simulink model "Hunt_crossley"  (Simulink 10.1)
settings: Solver=ode3  StartTime=0.0  StopTime=25  FixedStep=0.001  RelTol=1e-3  EnableMultiTasking=on
undefined symbols (not defined in the file): sigbuilder_block
libraries: simulink x3
settings Model: Creator=x  LastModifiedBy=pedram
settings DataIOCC: LimitDataPoints=on
settings OptimizationCC: ExpressionDepthLimit=2147483647
settings DebuggingCC: SolverPrmCheckMsg=warning  StateNameClashWarn=warning
settings GRTTargetCC: CombineOutputUpdateFcns=on  GRTInterface=off

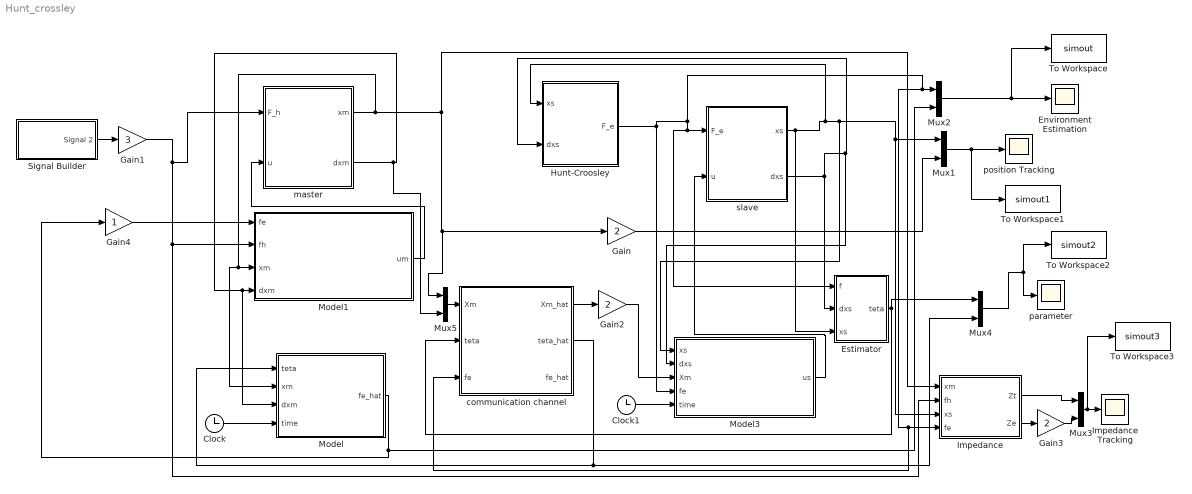
== system Hunt_crossley ==
  Clock : Clock
  Clock1 : Clock
  Environment Estimation : Scope
  Estimator : Subsystem
  Gain : Gain  Gain=2
  Gain1 : Gain  Gain=3
  Gain2 : Gain  Gain=2
  Gain3 : Gain  Gain=2
  Gain4 : Gain
  Hunt-Croosley : Subsystem
  Impedance : MATLAB Function  TreatAsAtomicUnit=on
  "Impedance Tracking " : Scope
  Model : MATLAB Function  TreatAsAtomicUnit=on
  Model1 : MATLAB Function  TreatAsAtomicUnit=on
  Model3 : MATLAB Function  TreatAsAtomicUnit=on
  Mux{1..5} (5 alike) : Mux  Inputs=2
  Signal Builder : Subsystem  Tag=STV Subsys  LoadFcn=sigbuilder_block('load');  StartFcn=sigbuilder_block('start');  StopFcn=sigbuilder_block('stop');  ClipboardFcn=sigbuilder_block('clipboard');  mask(Sigbuilder block){tuvar=[0:10]}
      mask help: Simulink:masks:SigbuilderBlock_MD
      mask init:
      | if ~strcmp(get_param(bdroot(gcbh),'SimulationStatus'),'stopped') tuvar = sigbuilder_block('maskInit'); end
      settings: CopyFcn=sigbuilder_block('copy');  DeleteFcn=sigbuilder_block('delete');  ModelCloseFcn=sigbuilder_block('modelClose');  PreSaveFcn=sigbuilder_block('preSave');  PauseFcn=sigbuilder_block('pause');  ContinueFcn=sigbuilder_block('continue');  NameChangeFcn=sigbuilder_block('namechange');  OpenFcn=sigbuilder_block('open',[216 34.1379 544.345 383.586 ]);  CloseFcn=sigbuilder_block('close');
      mask Display: plot(0, 0, 100, 100,[2, 2, 32, 32, 2], [68, 8, 8, 68, 68],[32, 2], [38, 38], [32, 19, 2],[53, 60, 44], [32, 17, 17, 2],[16, 16, 31, 31]);txt = getActiveGroup(gcbh);text(2, 100, txt,'verticalAlignment', 'top');
  To Workspace : ToWorkspace  VariableName=simout  SampleTime=-1
  To Workspace1 : ToWorkspace  VariableName=simout1  SampleTime=-1
  To Workspace2 : ToWorkspace  VariableName=simout2  SampleTime=-1
  To Workspace3 : ToWorkspace  VariableName=simout3  SampleTime=-1
  communication channel : Subsystem
  master : Subsystem
  parameter : Scope
  position Tracking : Scope
  slave : Subsystem
  wires:
  master/1(xm) -> Model/2(xm), Model1/3(xm), Mux5/1, Gain/1, Impedance/1(xm)
  slave/2(dxs) -> Model3/2(dxs), Hunt-Croosley/2(dxs), Estimator/2(dxs)
  Gain/1 -> Mux1/2
  Mux1/1 -> To Workspace1/1, position Tracking/1
  Impedance/1(Zt) -> Mux3/1
  Mux3/1 -> To Workspace3/1, "Impedance Tracking "/1
  communication channel/1(Xm_hat) -> Gain2/1
  Impedance/2(Ze) -> Gain3/1
  Signal Builder/1(Signal 2) -> Gain1/1
  Gain3/1 -> Mux3/2
  Model1/1(um) -> master/2(u)
  Model3/1(us) -> slave/2(u)
  master/2(dxm) -> Mux5/2, Model/3(dxm), Model1/4(dxm)
  Gain2/1 -> Model3/3(Xm)
  Clock/1 -> Model/4(time)
  communication channel/2(teta_hat) -> Model/1(teta), Mux4/2
  Estimator/1(teta) -> Mux4/1, communication channel/2(teta)
  Mux5/1 -> communication channel/1(Xm)
  Hunt-Croosley/1(F_e) -> slave/1(F_e), Estimator/1(f), communication channel/3(fe), Impedance/4(fe), Mux2/1, Model3/4(fe)
  Clock1/1 -> Model3/5(time)
  Mux2/1 -> To Workspace/1, Environment Estimation/1
  Mux4/1 -> To Workspace2/1, parameter/1
  Gain1/1 -> master/1(F_h), Model1/2(fh), Impedance/2(fh)
  slave/1(xs) -> Model3/1(xs), Impedance/3(xs), Mux1/1, Hunt-Croosley/1(xs), Estimator/3(xs)
  Model/1(fe_hat) -> Gain4/1, Mux2/2
  Gain4/1 -> Model1/1(fe)

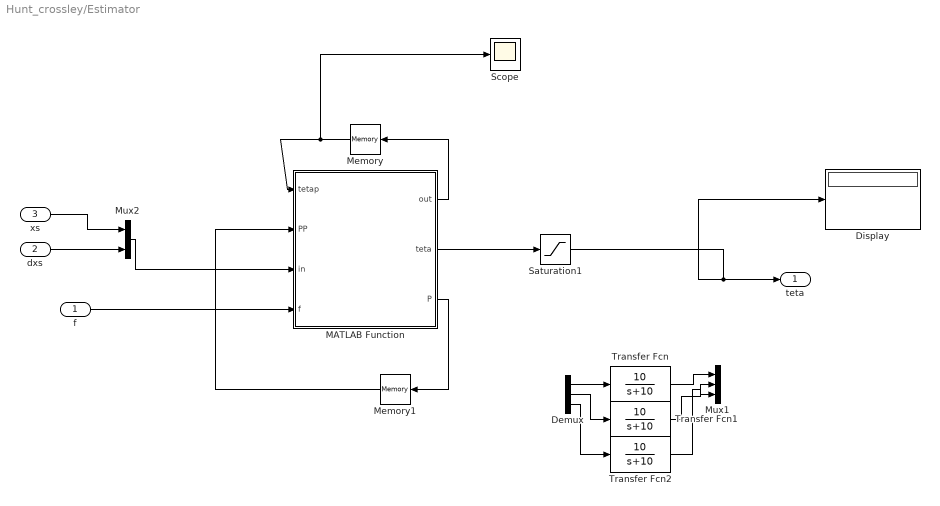
== system Hunt_crossley/Estimator ==
  f : Inport
  dxs : Inport  Port=2
  xs : Inport  Port=3
  Demux : Demux  Outputs=3
  Display : Display
  MATLAB Function : MATLAB Function  TreatAsAtomicUnit=on
  Memory : Memory  InitialCondition=[1;1;1]
  Memory1 : Memory  InitialCondition=10^2*eye(3,3)
  Mux1 : Mux  Inputs=3
  Mux2 : Mux  Inputs=2
  Saturation1 : Saturate  UpperLimit=5  LowerLimit=0
  Scope : Scope
  Transfer Fcn : TransferFcn  Numerator=[10]  Denominator=[1 10]
  Transfer Fcn1 : TransferFcn  Numerator=[10]  Denominator=[1 10]
  Transfer Fcn2 : TransferFcn  Numerator=[10]  Denominator=[1 10]
  teta : Outport
  wires:
  f/1 -> MATLAB Function/4(f)
  MATLAB Function/1(out) -> Memory/1
  Memory1/1 -> MATLAB Function/2(PP)
  Mux2/1 -> MATLAB Function/3(in)
  Memory/1 -> Scope/1, MATLAB Function/1(tetap)
  xs/1 -> Mux2/1
  dxs/1 -> Mux2/2
  MATLAB Function/3(P) -> Memory1/1
  Demux/1 -> Transfer Fcn/1
  Transfer Fcn/1 -> Mux1/1
  Transfer Fcn1/1 -> Mux1/2
  Transfer Fcn2/1 -> Mux1/3
  Demux/2 -> Transfer Fcn1/1
  Demux/3 -> Transfer Fcn2/1
  MATLAB Function/2(teta) -> Saturation1/1
  Saturation1/1 -> Display/1, teta/1

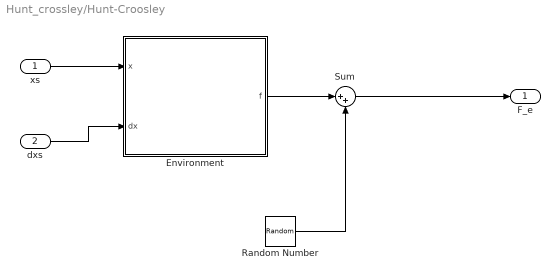
== system Hunt_crossley/Hunt-Croosley ==
  xs : Inport
  dxs : Inport  Port=2
  Environment : MATLAB Function  TreatAsAtomicUnit=on
  Random Number : RandomNumber  Variance=0.1
  Sum : Sum  Inputs=|++
  F_e : Outport
  wires:
  xs/1 -> Environment/1(x)
  dxs/1 -> Environment/2(dx)
  Environment/1(f) -> Sum/1
  Sum/1 -> F_e/1
  Random Number/1 -> Sum/2

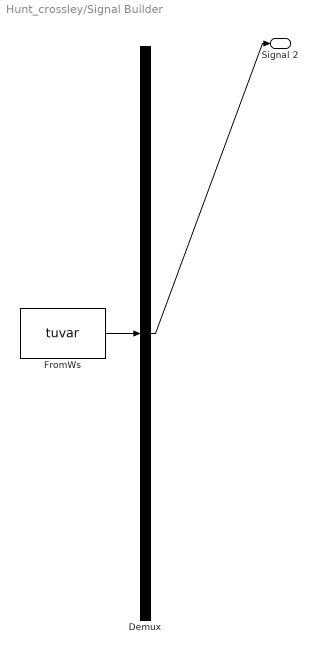
== system Hunt_crossley/Signal Builder ==
  Demux : Demux  Tag=STV Demux  Outputs=1
      settings: DisplayOption=none
  FromWs : FromWorkspace  Tag=STV FromWs  VariableName=tuvar  SigBuilderData=DataTag0  VnvData=DataTag1
      SigBuilderData=|
      | common.afterFinalStr = 'Extrapolate'
      | common.sampleTime = 0
      | dataSet.timeRange = [0 25]
      | dataSet.name = 'Group 1'
      | sbobj.Groups.Name = 'Group 1'
      | sbobj.Groups.Signals.Name = 'Signal 2'
      | sbobj.Groups.Signals.XData = [0 5.05 5.05 15.05 15.05 16.35 16.35 21.05 21.05 25]
      | sbobj.Groups.Signals.YData = [0.49 0.49 1.98 1.98 -0.82 -0.82 0.98 0.98 -0.24 -0.24]
      | sbobj.Groups.TimeRange = [0 25]
  Signal 2 : Outport  Tag=STV Outport
  wires:
  FromWs/1 -> Demux/1
  Demux/1 -> Signal 2/1

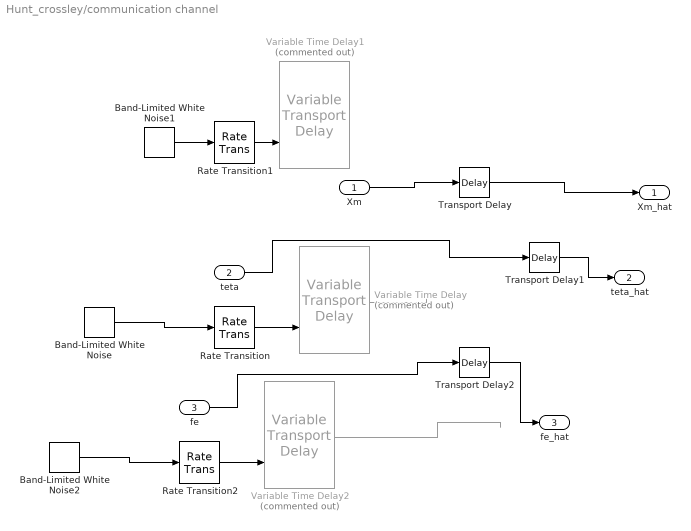
== system Hunt_crossley/communication channel ==
  Xm : Inport
  teta : Inport  Port=2
  fe : Inport  Port=3
  Band-Limited White Noise : simulink/Sources/Band-Limited White Noise  Cov=[0.1]  Ts=0.2  seed=[23341]
  Band-Limited White Noise1 : simulink/Sources/Band-Limited White Noise  Cov=[0.1]  Ts=0.2  seed=[5368541]
  Band-Limited White Noise2 : simulink/Sources/Band-Limited White Noise  Cov=[0.1]  Ts=0.2  seed=[28931]
  Rate Transition : RateTransition
  Rate Transition1 : RateTransition
  Rate Transition2 : RateTransition
  Transport Delay : TransportDelay
  Transport Delay1 : TransportDelay
  Transport Delay2 : TransportDelay
  Variable Time Delay : VariableTransportDelay  Commented=on  MaximumDelay=4  TransDelayFeedthrough=on
  Variable Time Delay1 : VariableTransportDelay  Commented=on  MaximumDelay=4  TransDelayFeedthrough=on
  Variable Time Delay2 : VariableTransportDelay  Commented=on  MaximumDelay=4  TransDelayFeedthrough=on
  Xm_hat : Outport
  teta_hat : Outport  Port=2
  fe_hat : Outport  Port=3
  wires:
  Band-Limited White Noise/1 -> Rate Transition/1
  Rate Transition/1 -> Variable Time Delay/2
  Band-Limited White Noise1/1 -> Rate Transition1/1
  Rate Transition1/1 -> Variable Time Delay1/2
  Variable Time Delay/1 -> ?
  Band-Limited White Noise2/1 -> Rate Transition2/1
  Rate Transition2/1 -> Variable Time Delay2/2
  Variable Time Delay2/1 -> ?
  fe/1 -> Transport Delay2/1
  Xm/1 -> Transport Delay/1
  Transport Delay/1 -> Xm_hat/1
  Transport Delay1/1 -> teta_hat/1
  teta/1 -> Transport Delay1/1
  Transport Delay2/1 -> fe_hat/1

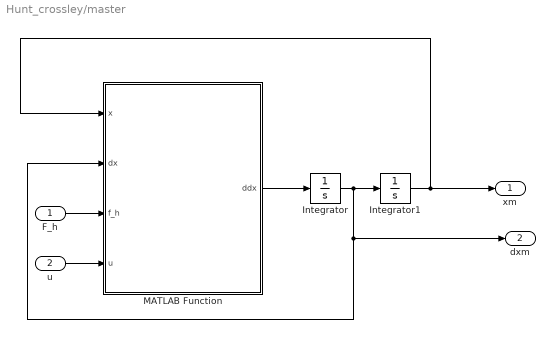
== system Hunt_crossley/master ==
  F_h : Inport
  u : Inport  Port=2
  Integrator : Integrator
  Integrator1 : Integrator
  MATLAB Function : MATLAB Function  TreatAsAtomicUnit=on
  xm : Outport
  dxm : Outport  Port=2
  wires:
  F_h/1 -> MATLAB Function/3(f_h)
  u/1 -> MATLAB Function/4(u)
  MATLAB Function/1(ddx) -> Integrator/1
  Integrator/1 -> dxm/1, MATLAB Function/2(dx), Integrator1/1
  Integrator1/1 -> MATLAB Function/1(x), xm/1

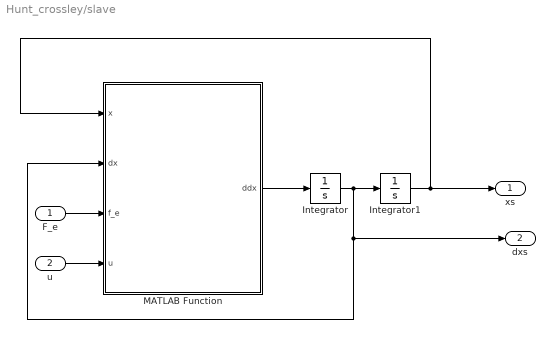
== system Hunt_crossley/slave ==
  F_e : Inport
  u : Inport  Port=2
  Integrator : Integrator
  Integrator1 : Integrator
  MATLAB Function : MATLAB Function  TreatAsAtomicUnit=on
  xs : Outport
  dxs : Outport  Port=2
  wires:
  F_e/1 -> MATLAB Function/3(f_e)
  u/1 -> MATLAB Function/4(u)
  MATLAB Function/1(ddx) -> Integrator/1
  Integrator/1 -> dxs/1, MATLAB Function/2(dx), Integrator1/1
  Integrator1/1 -> xs/1, MATLAB Function/1(x)

== matlab function slave/MATLAB Function ==
  data: x input double; dx input double; f_e input double; u input double; ddx output double
function ddx = fcn(x,dx,f_e,u)
%parameter
ms=0.07; bs=0.05;ks=0.08; 
ms=1; bs=0.5;ks=0.8; 

ddx=ms^-1*(u-f_e-bs*dx-ks*x);

== matlab function master/MATLAB Function ==
  data: x input double; dx input double; f_h input double; u input double; ddx output double
function ddx = fcn(x,dx,f_h,u)
%parameter
jm=0.05; bm=0.03;km=0.1; l_eff=0.5;

ddx=jm^-1*(u+f_h*l_eff-bm*dx-km*x);

== matlab function Estimator/MATLAB Function ==
  data: out output double; tetap input double; PP input double; in input double; f input double; teta output double; P output double
% function [out, teta, P]= fcn(tetap,   PP,   in,   f)
% parameter
% landa=1;
% if (in(1)<0.1 || f<0.1)
%    out=[1;1;1];
%    teta=[0;0;1];
%    P=10^3*eye(3,3);
% else
% phi=[1;in(2);log(in(1))];
% L=PP*phi/(landa+phi'*PP*phi);
% P=1/landa*(PP-L*phi'*PP);
% out=tetap+L*(log(f)-phi'*tetap);
% teta=[exp(out(1)); out(2)*exp(out(1));out(3)];
% if (P(1,1)>1000)
%     P(1,1)=1000;
% end
% if (P(2,2)>1000)
%      P(2,2)=1000;
% end
% if (P(3,3)>1000)
%      P(3,3)=1000;
% end
% end
% end
function [out, teta, P]= fcn(tetap,   PP,   in,   f)
%parameter
landa=1;
if (in(1)<0.1 || f<0.1)
   out=[1;1;1];
   teta=[0;0;1];
   P=10^3*eye(3,3);
else
phi=[1;in(2);log(in(1))];
L=PP*phi/(landa+phi'*PP*phi);
P=1/landa*(PP-L*phi'*PP);
out=tetap+L*(log(f)-phi'*tetap);
teta=[exp(out(1)); out(2)*exp(out(1));out(3)];
if (P(1,1)>1000)
    P(1,1)=1000;
end
if (P(2,2)>1000)
     P(2,2)=1000;
end
if (P(3,3)>1000)
     P(3,3)=1000;
end
end
end

== matlab function Impedance ==
  data: xm input double; fh input double; xs input double; Zt output double; fe input double; Ze output double
function [Zt,Ze] = impedance(xm,fh,xs,fe)
%control parameter
if xm<1e-3 && xm>-1e-3
    Zt=0;
else 
    Zt=fh/xm;
end
if xs<1e-3
   Ze=0;
else
    Ze=fe/xs;
end

== matlab function Hunt-Croosley/Environment ==
  data: x input double; dx input double; f output double
function f= ENV( x,dx )
%   Parameter
K=4;B=2.3; n=1.7;

if x<0
    f=0;
else
    f=(x^n)*(K+B*dx);
end

end

== matlab function Model ==
  data: teta input double; fe_hat output double; xm input double; dxm input double; time input double
function fe_hat= ENV_Model( teta ,xm,dxm,time)
%   Parameter
kp=2;
if time==0.001
fe_hat=0;
else
if xm<0
   fe_hat=0;
else
    K=teta(1);B=teta(2); n=teta(3);
    fe_hat=(kp*xm)^n*(K+B*(kp*dxm));
end
end
end

== matlab function Model1 ==
  data: fe input double; um output double; fh input double; xm input double; dxm input double
function um= Master_Impedance_control( fe,fh,xm,dxm )
%   Parameter
jm=0.05; bm=0.03;km=0.1; l_eff=0.5;
% jmd=0.6; bmd=4;kmd=2;
% 
% um=(bm-jm/jmd*bmd)*dxm+(km-jm/jmd*kmd)*xm+(jm/jmd)*(fh-fe)-l_eff*fh;

jmd=0.6*20; bmd=4*2;kmd=2*2;

um=(bm-jm/jmd*bmd)*dxm+(km-jm/jmd*kmd)*xm+(jm/jmd)*(fh-fe)-l_eff*fh;

end

== matlab function Model3 ==
  data: xs input double; dxs input double; Xm input double; fe input double; us output double; time input double
function us= slave_Impedance_control( xs,dxs,Xm,fe,time )
%   Parameter
ms=1; bs=0.5;ks=0.8; 
jsd=50; bsd=150;ksd=100;
if time==0.001
    us=0;
else
xm=Xm(1);
dxm=Xm(2);
us=-(ms/jsd*bsd)*(dxs-dxm)-(ms/jsd*ksd)*(xs-xm)+(1-0*ms/jsd)*fe+bs*dxs+ks*xs;
end
end
